simulink model "dc_model_advanced_control (2)"  (R2020b)
settings: Solver=VariableStepAuto  StartTime=0.0  StopTime=10.0  RelTol=1e-3
values from neighbouring files (symbols this model uses):
  J_m = 0.032    [HighWire_Artist_Dynamic_Model.m]    (also in llllllllllllllllllll.m; lqr_advanced_project.m; nnnnnnnn.m = 0.37)
  J_R = 0.0488    [HighWire_Artist_Dynamic_Model.m]    (also in llllllllllllllllllll.m; lqr_advanced_project.m; nnnnnnnn.m = 1.5)
  K_m = 0.0109    [HighWire_Artist_Dynamic_Model.m]    (also in llllllllllllllllllll.m; lqr_advanced_project.m; nnnnnnnn.m = 21)
  L = 0.1810    (= 0.181)    [HighWire_Artist_Dynamic_Model.m]    (also in llllllllllllllllllll.m; lqr_advanced_project.m; nnnnnnnn.m = 1.8)
  N = 14    [HighWire_Artist_Dynamic_Model.m]    (also in llllllllllllllllllll.m = 3; lqr_advanced_project.m = 0; nnnnnnnn.m = 1)
  R_m = 1.6    [HighWire_Artist_Dynamic_Model.m]    (also in llllllllllllllllllll.m; lqr_advanced_project.m; nnnnnnnn.m = 40)
settings Model: Creator=A family  LastModifiedBy=A family

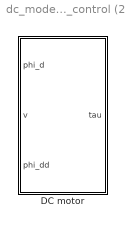
== system dc_model_advanced_control (2) ==
  DC motor : Subsystem
  wires:
  ? -> DC motor/2(v)

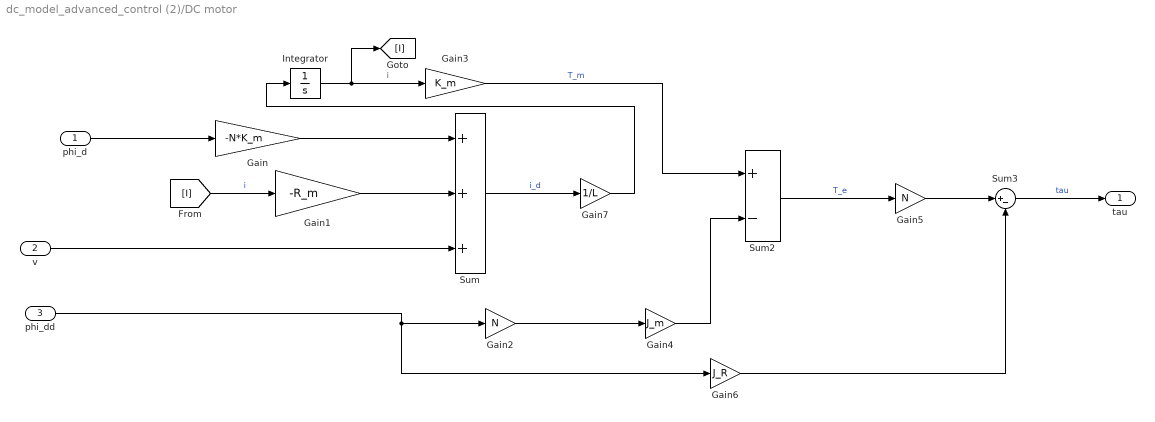
== system dc_model_advanced_control (2)/DC motor ==
  phi_d : Inport
  v : Inport  Port=2
  phi_dd : Inport  Port=3
  Gain : Gain  Gain=-N*K_m
  Gain1 : Gain  Gain=-R_m
  Gain2 : Gain  Gain=N
  Gain3 : Gain  Gain=K_m
  Gain4 : Gain  Gain=J_m
  Gain5 : Gain  Gain=N
  Gain6 : Gain  Gain=J_R
  Gain7 : Gain  Gain=1/L
  Integrator : Integrator
  Sum : Sum  Inputs=+++
  Sum2 : Sum  Inputs=+-
  Sum3 : Sum  Inputs=|+-
  tau : Outport
  wires:
  Gain1/1 -> Sum/2
  Gain2/1 -> Gain4/1
  Gain6/1 -> Sum3/2
  Gain/1 -> Sum/1
  phi_dd/1 -> Gain6/1, Gain2/1
  Sum/1 -> Gain7/1  "i_d"
  Integrator/1 -> [I], Gain3/1  "i"
  Gain4/1 -> Sum2/2
  Gain5/1 -> Sum3/1
  Sum3/1 -> tau/1  "tau"
  phi_d/1 -> Gain/1
  Sum2/1 -> Gain5/1  "T_e"
  v/1 -> Sum/3
  Gain3/1 -> Sum2/1  "T_m"
  [I] -> Gain1/1  "i"
  Gain7/1 -> Integrator/1
